simulink model "Sim_pH1"  (R2018a)
settings: Solver=ode45  StartTime=0.0  StopTime=5000  RelTol=1e-3  EnableMultiTasking=on
settings Model: Creator=NIFEMI  LastModifiedBy=Owolabi Israel
settings SolverCC: AlgebraicLoopSolver=LineSearch
settings DataIOCC: LimitDataPoints=on  SaveFormat=Array
settings OptimizationCC: LifeSpan=inf
settings DebuggingCC: SolverPrmCheckMsg=warning  SFUnexpectedBacktrackingDiag=warning  SFNoUnconditionalDefaultTransitionDiag=warning  SFExecutionAtInitializationDiag=none
settings HardwareCC: ProdBitPerPointer=32  ProdBitPerSizeT=32  ProdBitPerPtrDiffT=32  ProdLargestAtomicFloat=None  ProdIntDivRoundTo=Undefined  ProdEndianess=Unspecified  ProdWordSize=32  ProdHWDeviceType=32-bit Generic
settings ModelReferenceCC: PropagateSignalLabelsOutOfModel=off
settings CodeAppCC: StateflowObjectComments=on
settings GRTTargetCC: TargetLangStandard=C89/C90 (ANSI)  GeneratePreprocessorConditionals=Disable all
settings ConfigComp: CovMetricSettings=dw  CovHtmlReporting=on  CovSaveCumulativeToWorkspaceVar=on  CovSaveSingleToWorkspaceVar=on  CovExternalEMLEnable=off  CovSFcnEnable=off

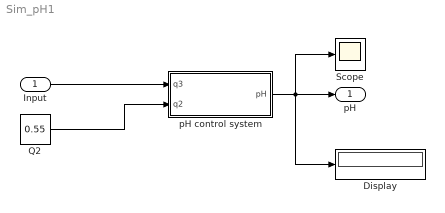
== system Sim_pH1 ==
  Input : Inport
  Display : Display
  Q2 : Constant  Value=0.55
  Scope : Scope
  pH control system : Subsystem
  pH : Outport
  wires:
  Input/1 -> pH control system/1(q3)
  pH control system/1(pH) -> Scope/1, Display/1, pH/1
  Q2/1 -> pH control system/2(q2)

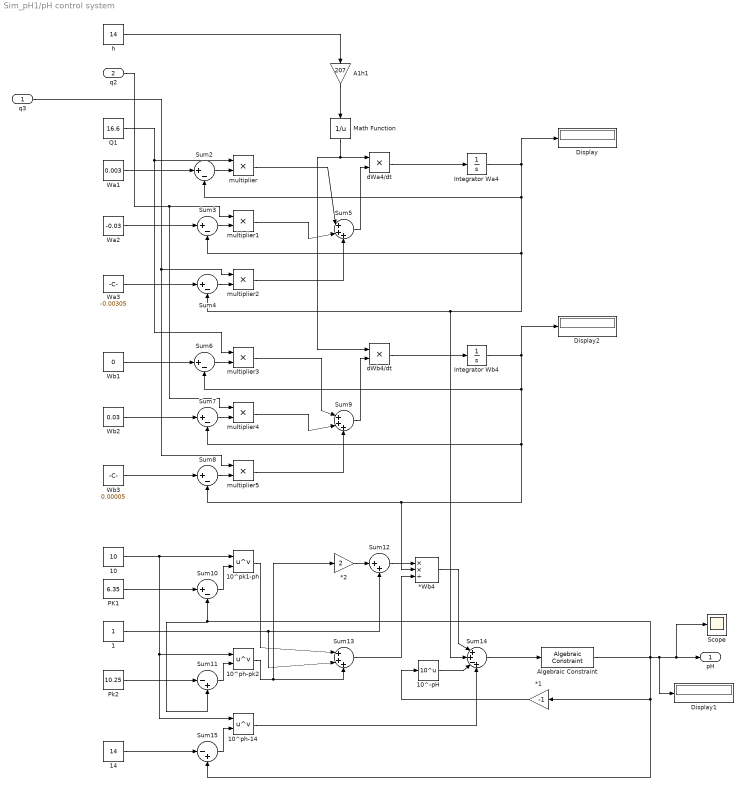
== system Sim_pH1/pH control system ==
  q3 : Inport
  q2 : Inport  Port=2
  *1 : Gain  Gain=-1
  *2 : Gain  Gain=2
  *Wb4 : Product  Inputs=**/
  1 : Constant
  10 : Constant  Value=10
  10^-pH : Math  Operator=10^u  SaturateOnIntegerOverflow=on
  10^ph-14 : Math  Operator=pow  SaturateOnIntegerOverflow=on
  10^ph-pk2 : Math  Operator=pow  SaturateOnIntegerOverflow=on
  10^pk1-ph : Math  Operator=pow  SaturateOnIntegerOverflow=on
  14 : Constant  Value=14
  A1h1 : Gain  Gain=207
  Algebraic Constraint : AlgebraicConstraint  InitialGuess=7
  Display : Display
  Display1 : Display
  Display2 : Display
  Integrator Wa4 : Integrator  InitialCondition=-0.000432
  Integrator Wb4 : Integrator  InitialCondition=0.000528
  Math Function : Math  Operator=reciprocal  SaturateOnIntegerOverflow=on
  PK1 : Constant  Value=6.35
  Pk2 : Constant  Value=10.25
  Q1 : Constant  Value=16.6
  Scope : Scope
  Sum{2..4,6..8,10} (7 alike) : Sum  Inputs=|+-
  Sum11 : Sum  Inputs=|-+
  Sum12 : Sum  Inputs=|++
  Sum13 : Sum  Inputs=|+++
  Sum14 : Sum  Inputs=|++-+
  Sum15 : Sum  Inputs=|-+
  Sum5 : Sum  Inputs=|+++
  Sum9 : Sum  Inputs=|+++
  Wa1 : Constant  Value=0.003
  Wa2 : Constant  Value=-0.03
  Wa3 : Constant  Value=-0.00305
  Wb1 : Constant  Value=0
  Wb2 : Constant  Value=0.03
  Wb3 : Constant  Value=0.00005
  dWa4/dt : Product
  dWb4/dt : Product
  h : Constant  Value=14
  multiplier{,1..5} (6 alike) : Product
  pH : Outport
  wires:
  Sum4/1 -> multiplier2/2
  Wa2/1 -> Sum3/1
  Sum7/1 -> multiplier4/2
  dWb4/dt/1 -> Integrator Wb4/1
  Integrator Wa4/1 -> Display/1, Sum2/2, Sum3/2, Sum14/2, Sum4/2
  Sum2/1 -> multiplier/2
  10^pk1-ph/1 -> Sum13/1
  q2/1 -> multiplier4/1, multiplier1/1
  Sum9/1 -> dWb4/dt/2
  multiplier1/1 -> Sum5/2
  h/1 -> A1h1/1
  dWa4/dt/1 -> Integrator Wa4/1
  Sum6/1 -> multiplier3/2
  *Wb4/1 -> Sum14/1
  multiplier/1 -> Sum5/1
  Algebraic Constraint/1 -> Sum11/2, Sum10/2, Display1/1, Scope/1, pH/1, *1/1, Sum15/2
  Q1/1 -> multiplier3/1, multiplier/1
  10^ph-pk2/1 -> *2/1, Sum13/3
  multiplier5/1 -> Sum9/3
  Integrator Wb4/1 -> Display2/1, Sum6/2, Sum7/2, *Wb4/2, Sum8/2
  A1h1/1 -> Math Function/1
  Wa3/1 -> Sum4/1
  multiplier2/1 -> Sum5/3
  10/1 -> 10^ph-pk2/1, 10^ph-14/1, 10^pk1-ph/1
  Sum14/1 -> Algebraic Constraint/1
  Pk2/1 -> Sum11/1
  Sum13/1 -> *Wb4/3
  PK1/1 -> Sum10/1
  Sum12/1 -> *Wb4/1
  Sum11/1 -> 10^ph-pk2/2
  10^-pH/1 -> Sum14/3
  Sum10/1 -> 10^pk1-ph/2
  1/1 -> Sum13/2, Sum12/2
  Math Function/1 -> dWa4/dt/1, dWb4/dt/1
  Wb2/1 -> Sum7/1
  *1/1 -> 10^-pH/1
  10^ph-14/1 -> Sum14/4
  multiplier3/1 -> Sum9/1
  Wb1/1 -> Sum6/1
  *2/1 -> Sum12/1
  Sum8/1 -> multiplier5/2
  Wa1/1 -> Sum2/1
  q3/1 -> multiplier5/1, multiplier2/1
  multiplier4/1 -> Sum9/2
  Wb3/1 -> Sum8/1
  Sum5/1 -> dWa4/dt/2
  14/1 -> Sum15/1
  Sum3/1 -> multiplier1/2
  Sum15/1 -> 10^ph-14/2
